simulink model "attitude_modela"  (R2021a)
settings: Solver=VariableStepAuto  StartTime=0.0  StopTime=2000  MaxStep=200
InitFcn:
  | run('parameters.m')
StartFcn:
  | run('parameters.m')
values from neighbouring files (symbols this model uses):
  ARW = (1/4*deg2rad([0.2 0.2 0.2]/sqrt(3600))).^2    [parameters.m]
  c_gyro = 2*sqrt(k*Jz)    [parameters.m]
  Ir = 1e-2    (= 0.01)    [parameters.m]
  J = [0.09 0 0; 0 0.14 0; 0 0 0.07]    [parameters.m]
  Jz = 2e-2    (= 0.02)    [parameters.m]
  k = 10    [parameters.m]    (also in prova.m = size(IGRF,1))
  m_par = [.1 .1 .1]    [parameters.m]
  mu = 398600    [parameters.m]
  nt0 = 0    [parameters.m]
  par = [40073 e deg2rad(59.2548) deg2rad(50) deg2rad(280)]    [parameters.m]
  RRW = (1/4*deg2rad([0.3 0.3 0.3]/3600)).^2    [parameters.m]
  Sch =     [IGRF.mat]
  tsg = 1e-1    (= 0.1)    [parameters.m]
  wr = 100*pi/180    (= 1.74532925199)    [parameters.m]
undefined symbols (not defined in the file or in its folder): DiscIntNeverNeededParam, solar_par
libraries: dspmathops x1, pid_lib x1
settings Model: Creator=matte  LastModifiedBy=simon

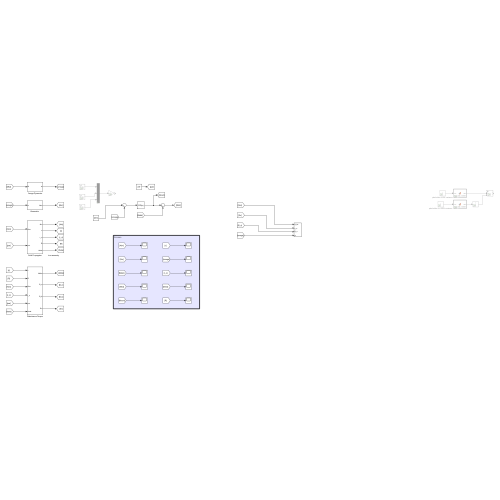
[thumbnail: Simulink's stored preview of the top-level diagram]
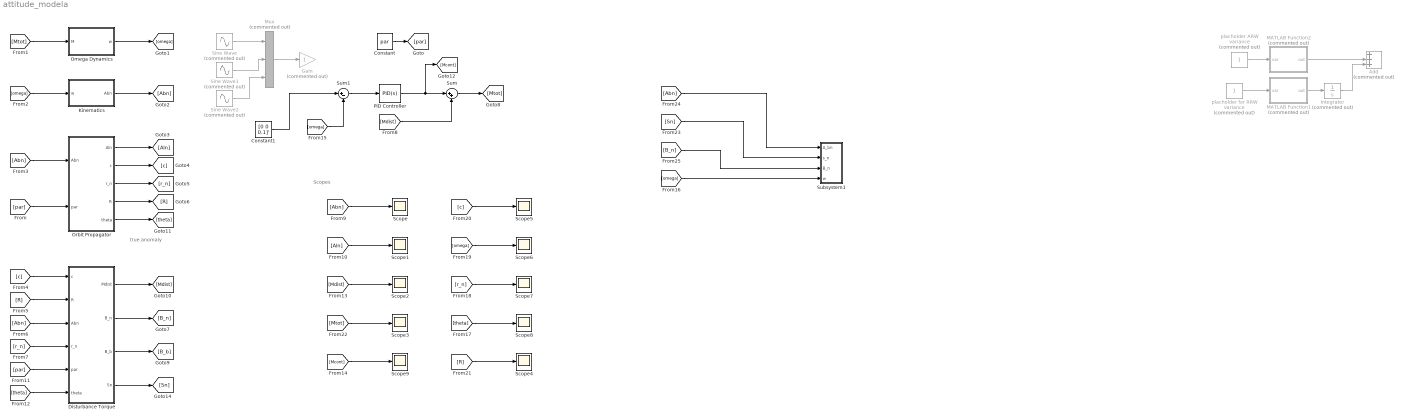
== system attitude_modela ==
  note: Scopes
  note: true anomaly
  Add : Sum  Commented=on  Inputs=+++
  Constant : Constant  Value=par
  Constant1 : Constant  Value=[0 0 0.1]'
  Disturbance Torque : Subsystem
  Gain : Gain  Commented=on
  Integrator : Integrator  Commented=on
  Kinematics : Subsystem
  MATLAB Function1 : MATLAB Function  Commented=on  TreatAsAtomicUnit=on
  MATLAB Function2 : MATLAB Function  Commented=on  TreatAsAtomicUnit=on
  Mux : Mux  Commented=on  Inputs=3
  Omega Dynamics : Subsystem
  Orbit Propagator : Subsystem
  PID Controller : pid_lib/PID Controller  Controller=PID  Form=Parallel  TimeDomain=Continuous-time  UseExternalTs=off  SampleTime=-1  IntegratorMethod=Forward Euler  FilterMethod=Forward Euler  ControllerParametersSource=internal  P=0.1  I=0.01  D=0  UseFilter=on  N=100  TunerSelectOption=Transfer Function Based (PID Tuner App)  InitialConditionSource=internal  InitialConditionForIntegrator=0  InitialConditionForFilter=0  DifferentiatorICPrevScaledInput=0  ExternalReset=none  TrackingMode=off  Kt=1  LimitOutput=off  SatLimitsSource=internal  UpperSaturationLimit=inf  LowerSaturationLimit=-inf  LinearizeAsGain=on  AntiWindupMode=none  Kb=1  POutMin=[]  POutMax=[]  IOutMin=[]  IOutMax=[]  DOutMin=[]  DOutMax=[]  NOutMin=[]  NOutMax=[]  SumOutMin=[]  SumOutMax=[]  SaturationOutMin=[]  SaturationOutMax=[]  PParamMin=[]  PParamMax=[]  IParamMin=[]  IParamMax=[]  DParamMin=[]  DParamMax=[]  NParamMin=[]  NParamMax=[]  KbParamMin=[]  KbParamMax=[]  KtParamMin=[]  KtParamMax=[]  KbOutMin=[]  KbOutMax=[]  KtOutMin=[]  KtOutMax=[]  IntegratorOutMin=[]  IntegratorOutMax=[]  FilterOutMin=[]  FilterOutMax=[]  SumI1OutMin=[]  SumI1OutMax=[]  SumI2OutMin=[]  SumI2OutMax=[]  SumI3OutMin=[]  SumI3OutMax=[]  SumI4OutMin=[]  SumI4OutMax=[]  SumDOutMin=[]  SumDOutMax=[]  DifferentiatorOutMin=[]  DifferentiatorOutMax=[]  FilterDiffOutCoefMin=[]  FilterDiffOutCoefMax=[]  ReciprocalOutMin=[]  ReciprocalOutMax=[]  SumDenOutMin=[]  SumDenOutMax=[]  SumNumOutMin=[]  SumNumOutMax=[]  DivideOutMin=[]  DivideOutMax=[]  UdiffTsProdOutMin=[]  UdiffTsProdOutMax=[]  NTsProdOutMin=[]  NTsProdOutMax=[]  UintegralTsProdOutMin=[]  UintegralTsProdOutMax=[]  UngainTsProdOutMin=[]  UngainTsProdOutMax=[]  IntegratorContinuousStateAttributes=''  IntegratorStateMustResolveToSignalObject=off  IntegratorRTWStateStorageClass=Auto  FilterContinuousStateAttributes=''  FilterStateMustResolveToSignalObject=off  FilterRTWStateStorageClass=Auto  ParallelPVariant=InternalParameters  IdealPVariant=Disabled  IVariant=InternalParameters  DVariant=InternalParameters  IntegratorVariant=Continuous  SatVariant=Disabled  AWVariant=Passthrough  PCopyVariant=Disabled  TRVariant=Disabled  FdbkBlocksVariant=Forward  IdealPFdbkVariant=Disabled  SatFdbkVariant=Disabled  DerivativeFilterVariant=ContFilter  NVariant=InternalParameters  NCopyVariant=Disabled  FilterICVariant=InternalICsFilter  IntegratorICVariant=InternalICs  ExternalResetVariant=Disabled  TRSumVariant=Passthrough  SumFdbkVariant=Disabled  SumVariant=Sum_PID  TsampFilterVariant=InternalTs  TsampNgainVariant=Passthrough  TsampIntegralVariant=Passthrough  ExternalSaturationOutDataTypeStr=Inherit: Same as second input
  Scope{,1..9} (10 alike) : Scope
  Sine Wave : Sin  Commented=on  Amplitude=3  Frequency=2*pi*1e-3  SampleTime=0
  Sine Wave1 : Sin  Commented=on  Amplitude=0.5  Frequency=2*pi*5e-4*0  SampleTime=0
  Sine Wave2 : Sin  Commented=on  Amplitude=0.01  Frequency=2*pi*1e-3  SampleTime=0
  Subsystem1 : Subsystem
  Sum : Sum  Inputs=|++
  Sum1 : Sum  Inputs=|+-
  placholder ARW variance : Constant  Commented=on
  placholder for RRW variance : Constant  Commented=on
  wires:
  Constant/1 -> [par]
  [par] -> Orbit Propagator/2(par)
  PID Controller/1 -> [Mcont], Sum/1
  [Mtot] -> Omega Dynamics/1(M)
  Omega Dynamics/1(w) -> [omega]
  [omega] -> Kinematics/1(w)
  Kinematics/1(Abn) -> [Abn]
  [Abn] -> Orbit Propagator/1(Abn)
  Orbit Propagator/4(R) -> [R]
  Orbit Propagator/3(r_n) -> [r_n]
  Orbit Propagator/2(c) -> [c]
  Orbit Propagator/1(Aln) -> [Aln]
  [Mdist] -> Sum/2
  Sum/1 -> [Mtot]
  Orbit Propagator/5(theta) -> [theta]
  [c] -> Disturbance Torque/1(c)
  [R] -> Disturbance Torque/2(R)
  [Abn] -> Disturbance Torque/3(Abn)
  [r_n] -> Disturbance Torque/4(r_n)
  [par] -> Disturbance Torque/5(par)
  [theta] -> Disturbance Torque/6(theta)
  Disturbance Torque/1(Mdist) -> [Mdist]
  [Abn] -> Scope/1
  [Mdist] -> Scope2/1
  [R] -> Scope4/1
  [omega] -> Scope6/1
  [theta] -> Scope8/1
  [r_n] -> Scope7/1
  [c] -> Scope5/1
  [Mtot] -> Scope3/1
  [Aln] -> Scope1/1
  Disturbance Torque/2(B_n) -> [B_n]
  Disturbance Torque/3(B_b) -> [B_b]
  [Mcont] -> Scope9/1
  MATLAB Function1/1(out) -> Integrator/1
  Integrator/1 -> Add/3
  MATLAB Function2/1(out) -> Add/2
  placholder ARW variance/1 -> MATLAB Function2/1(var)
  placholder for RRW variance/1 -> MATLAB Function1/1(var)
  Disturbance Torque/4(Sn) -> [Sn]
  [omega] -> Sum1/2
  Sum1/1 -> PID Controller/1
  Sine Wave/1 -> Mux/1
  Sine Wave1/1 -> Mux/2
  Sine Wave2/1 -> Mux/3
  Mux/1 -> Gain/1
  [Abn] -> Subsystem1/1(A_bn)
  [Sn] -> Subsystem1/2(s_n)
  [B_n] -> Subsystem1/3(B_n)
  [omega] -> Subsystem1/4(w)
  Constant1/1 -> Sum1/1

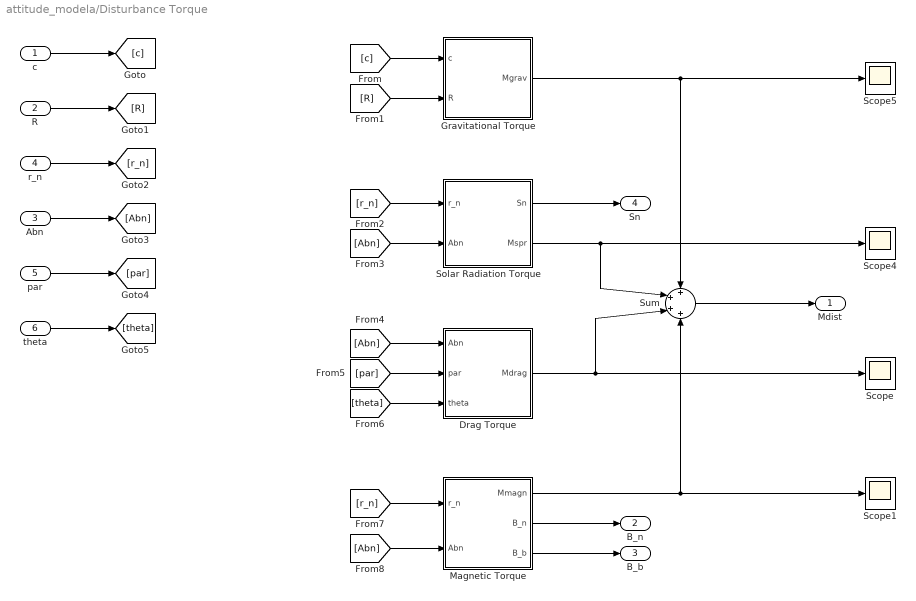
== system attitude_modela/Disturbance Torque ==
  c : Inport
  R : Inport  Port=2
  Abn : Inport  Port=3
  r_n : Inport  Port=4
  par : Inport  Port=5
  theta : Inport  Port=6
  Drag Torque : Subsystem
  Gravitational Torque : Subsystem
  Magnetic Torque : Subsystem
  Scope{,1,4..5} (4 alike) : Scope
  Solar Radiation Torque : Subsystem
  Sum : Sum  Inputs=4
  Mdist : Outport
  B_n : Outport  Port=2
  B_b : Outport  Port=3
  Sn : Outport  Port=4
  wires:
  Sum/1 -> Mdist/1
  Magnetic Torque/2(B_n) -> B_n/1
  Magnetic Torque/3(B_b) -> B_b/1
  c/1 -> [c]
  R/1 -> [R]
  r_n/1 -> [r_n]
  Abn/1 -> [Abn]
  par/1 -> [par]
  theta/1 -> [theta]
  Magnetic Torque/1(Mmagn) -> Scope1/1, Sum/4
  Drag Torque/1(Mdrag) -> Sum/3, Scope/1
  Solar Radiation Torque/2(Mspr) -> Scope4/1, Sum/2
  Gravitational Torque/1(Mgrav) -> Scope5/1, Sum/1
  [Abn] -> Magnetic Torque/2(Abn)
  [r_n] -> Magnetic Torque/1(r_n)
  [Abn] -> Drag Torque/1(Abn)
  [par] -> Drag Torque/2(par)
  [theta] -> Drag Torque/3(theta)
  [Abn] -> Solar Radiation Torque/2(Abn)
  [r_n] -> Solar Radiation Torque/1(r_n)
  [R] -> Gravitational Torque/2(R)
  [c] -> Gravitational Torque/1(c)
  Solar Radiation Torque/1(Sn) -> Sn/1

== system attitude_modela/Kinematics ==
  w : Inport
  Gain : Gain  Gain=-1
  Integrator : Integrator  InitialCondition=eye(3)
  Levi-Civita Matrix : Subsystem
  Product : Product  Multiplication=Matrix(*)
  Subsystem : Subsystem
  Abn : Outport
  wires:
  Product/1 -> Gain/1
  Levi-Civita Matrix/1(w^) -> Product/1
  w/1 -> Levi-Civita Matrix/1(w)
  Gain/1 -> Integrator/1  "dA"
  Integrator/1 -> Subsystem/1(A0)
  Subsystem/1(A) -> Abn/1, Product/2

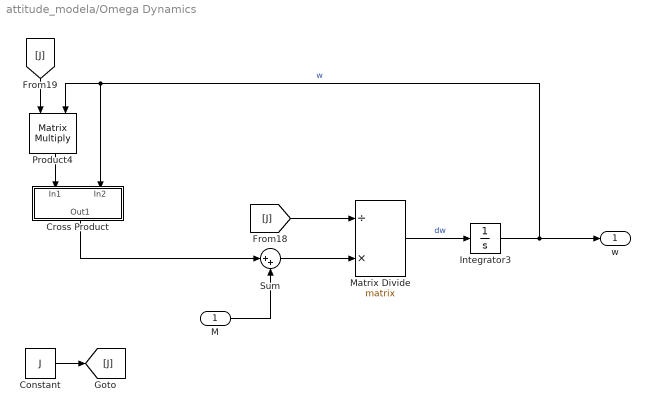
== system attitude_modela/Omega Dynamics ==
  M : Inport
  Constant : Constant  Value=J
  Cross Product : Subsystem  Description=Replaced Block  mask(Replaced Block){}
      mask help: This block has been replaced with an empty subsystem because it used functionality that is unavailable in Simulink R2021a.
      mask Display: fprintf('Replaced: %s\n','CrossProduct')
  Integrator3 : Integrator  InitialCondition=zeros(3,1)
  Matrix Divide : Product  Inputs=/*  Multiplication=Matrix(*)
  Product4 : Product  Multiplication=Matrix(*)
  Sum : Sum  Inputs=|++
  w : Outport
  wires:
  M/1 -> Sum/2
  Matrix Divide/1 -> Integrator3/1  "dw"
  Product4/1 -> Cross Product/1(In1)
  Integrator3/1 -> w/1, Product4/2, Cross Product/2(In2)  "w"
  Constant/1 -> [J]
  [J] -> Matrix Divide/1
  [J] -> Product4/1
  Cross Product/1(Out1) -> Sum/1
  Sum/1 -> Matrix Divide/2

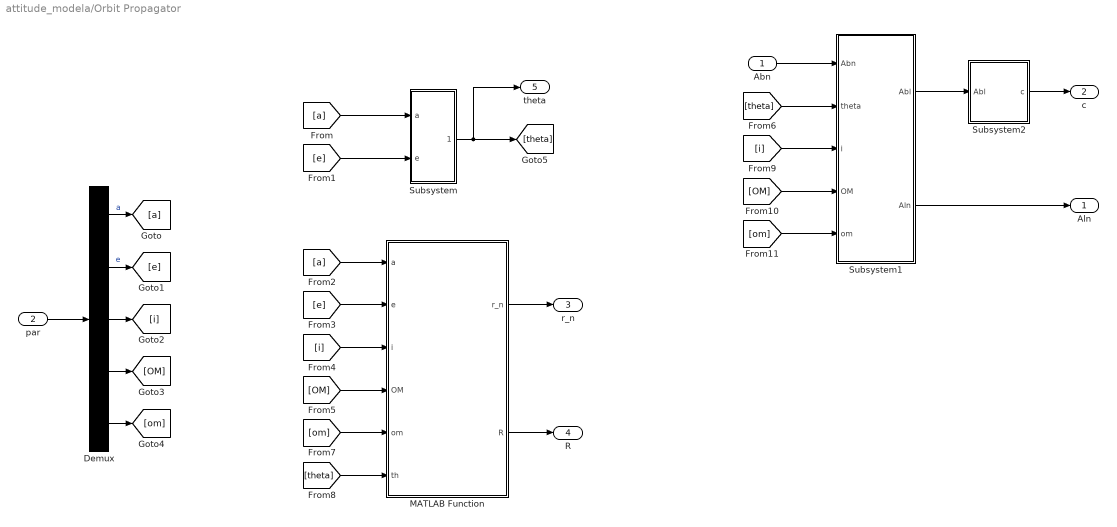
== system attitude_modela/Orbit Propagator ==
  Abn : Inport
  par : Inport  Port=2
  Demux : Demux  Outputs=5
  MATLAB Function : MATLAB Function  TreatAsAtomicUnit=on
  Subsystem : Subsystem
  Subsystem1 : Subsystem
  Subsystem2 : Subsystem
  Aln : Outport
  c : Outport  Port=2
  r_n : Outport  Port=3
  R : Outport  Port=4
  theta : Outport  Port=5
  wires:
  Abn/1 -> Subsystem1/1(Abn)
  Subsystem1/1(Abl) -> Subsystem2/1(Abl)
  Subsystem1/2(Aln) -> Aln/1
  par/1 -> Demux/1
  Subsystem2/1(c) -> c/1
  Demux/1 -> [a]  "a"
  Demux/2 -> [e]  "e"
  Demux/3 -> [i]
  Demux/4 -> [OM]
  Demux/5 -> [om]
  [e] -> MATLAB Function/2(e)
  [a] -> MATLAB Function/1(a)
  [OM] -> MATLAB Function/4(OM)
  [i] -> MATLAB Function/3(i)
  [theta] -> Subsystem1/2(theta)
  Subsystem/1(theta) -> theta/1, [theta]
  [om] -> MATLAB Function/5(om)
  [theta] -> MATLAB Function/6(th)
  MATLAB Function/1(r_n) -> r_n/1
  MATLAB Function/2(R) -> R/1
  [i] -> Subsystem1/3(i)
  [OM] -> Subsystem1/4(OM)
  [om] -> Subsystem1/5(om)
  [e] -> Subsystem/2(e)
  [a] -> Subsystem/1(a)

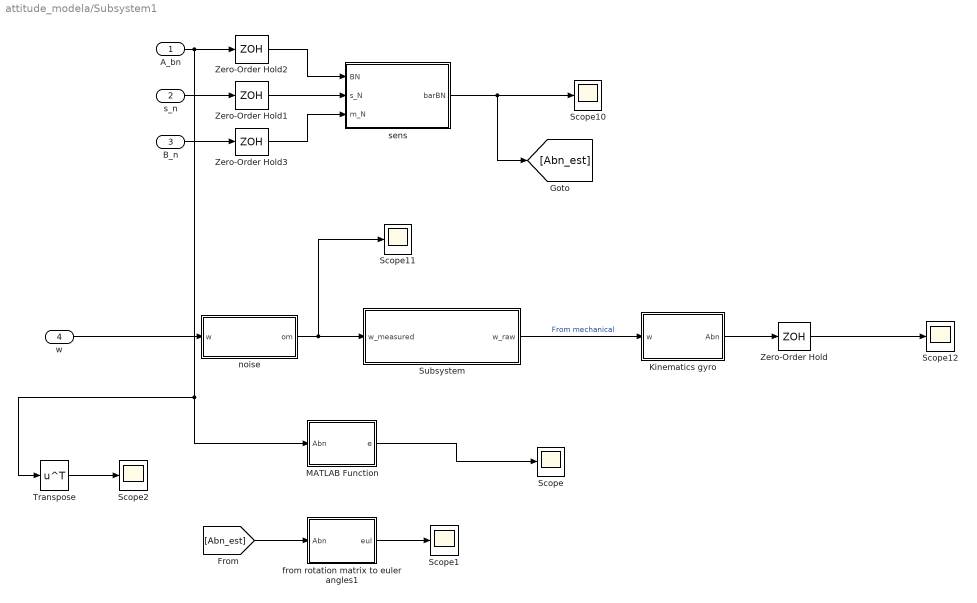
== system attitude_modela/Subsystem1 ==
  A_bn : Inport
  s_n : Inport  Port=2
  B_n : Inport  Port=3
  w : Inport  Port=4
  Kinematics gyro : Subsystem
  MATLAB Function : MATLAB Function  TreatAsAtomicUnit=on
  Scope{,1..2,10..12} (6 alike) : Scope
  Subsystem : Subsystem
  Transpose : Math  Operator=transpose  SaturateOnIntegerOverflow=on
  Zero-Order Hold{,1..3} (4 alike) : ZeroOrderHold  SampleTime=tsg
  from rotation matrix to euler angles1 : MATLAB Function  TreatAsAtomicUnit=on
  noise : Subsystem
  sens : MATLAB Function  TreatAsAtomicUnit=on
  wires:
  Zero-Order Hold/1 -> Scope12/1
  B_n/1 -> Zero-Order Hold3/1
  Kinematics gyro/1(Abn) -> Zero-Order Hold/1
  Subsystem/1(w_raw) -> Kinematics gyro/1(w)  "From mechanical"
  Zero-Order Hold1/1 -> sens/2(s_N)
  noise/1(om) -> Scope11/1, Subsystem/1(w_measured)
  Zero-Order Hold3/1 -> sens/3(m_N)
  sens/1(barBN) -> [Abn_est], Scope10/1
  w/1 -> noise/1(w)
  s_n/1 -> Zero-Order Hold1/1
  A_bn/1 -> Transpose/1, MATLAB Function/1(Abn), Zero-Order Hold2/1
  Zero-Order Hold2/1 -> sens/1(BN)
  [Abn_est] -> from rotation matrix to euler angles1/1(Abn)
  from rotation matrix to euler angles1/1(eul) -> Scope1/1
  MATLAB Function/1(e) -> Scope/1
  Transpose/1 -> Scope2/1

== system attitude_modela/Disturbance Torque/Drag Torque ==
  Abn : Inport
  par : Inport  Port=2
  theta : Inport  Port=3
  Drag Torque : MATLAB Function  TreatAsAtomicUnit=on
  Mdrag : Outport
  wires:
  Drag Torque/1(Mdrag) -> Mdrag/1
  Abn/1 -> Drag Torque/1(Abn)
  theta/1 -> Drag Torque/3(theta)
  par/1 -> Drag Torque/2(par)

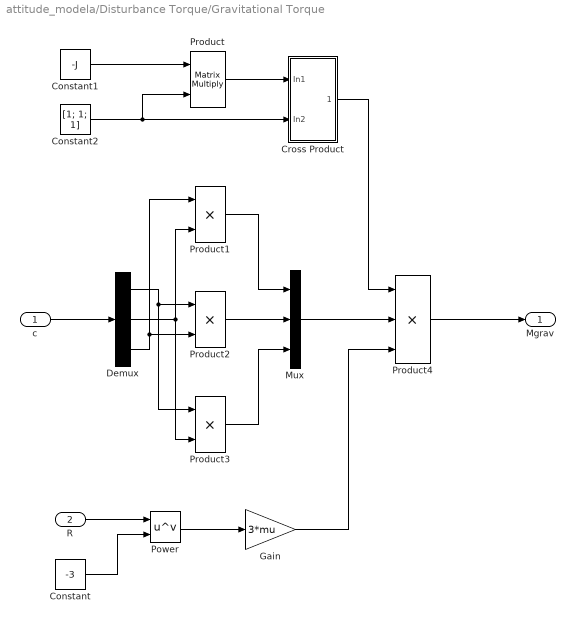
== system attitude_modela/Disturbance Torque/Gravitational Torque ==
  c : Inport
  R : Inport  Port=2
  Constant : Constant  Value=-3
  Constant1 : Constant  Value=-J
  Constant2 : Constant  Value=[1; 1; 1]
  Cross Product : Subsystem  Description=Replaced Block  mask(Replaced Block){}
      mask help: This block has been replaced with an empty subsystem because it used functionality that is unavailable in Simulink R2021a.
      mask Display: fprintf('Replaced: %s\n','CrossProduct')
  Demux : Demux  Outputs=3
  Gain : Gain  Gain=3*mu
  Mux : Mux  Inputs=3
  Power : Math  Operator=pow  SaturateOnIntegerOverflow=on
  Product : Product  Multiplication=Matrix(*)
  Product1 : Product
  Product2 : Product
  Product3 : Product
  Product4 : Product  Inputs=3
  Mgrav : Outport
  wires:
  Constant/1 -> Power/2
  R/1 -> Power/1
  Power/1 -> Gain/1
  Constant1/1 -> Product/1
  Constant2/1 -> Product/2, Cross Product/2(In2)
  Product/1 -> Cross Product/1(In1)
  c/1 -> Demux/1
  Demux/1 -> Product2/1, Product3/1
  Demux/3 -> Product1/1, Product2/2
  Demux/2 -> Product1/2, Product3/2
  Product2/1 -> Mux/2
  Product1/1 -> Mux/1
  Product3/1 -> Mux/3
  Cross Product/1(Out1) -> Product4/1
  Mux/1 -> Product4/2
  Gain/1 -> Product4/3
  Product4/1 -> Mgrav/1

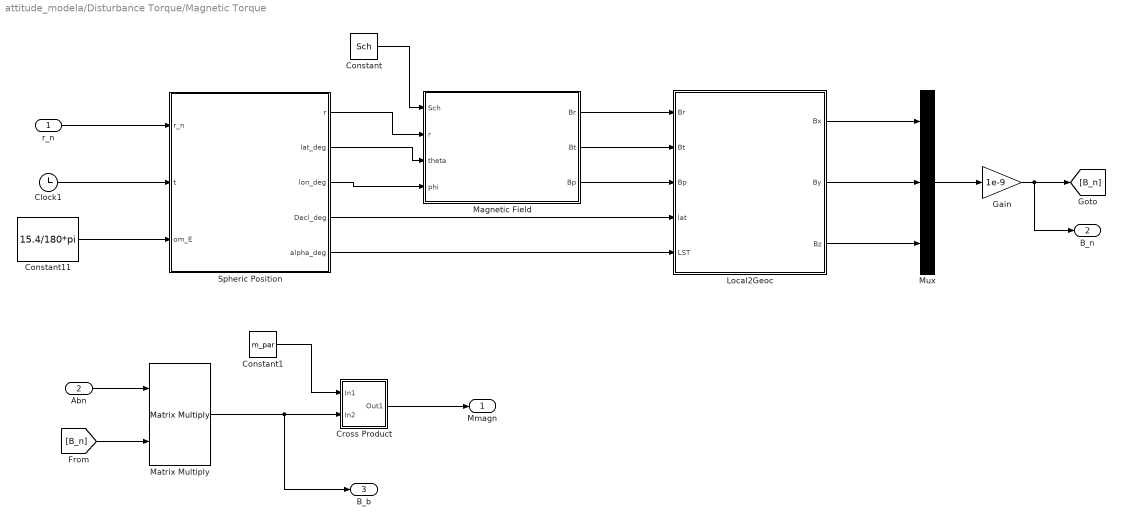
== system attitude_modela/Disturbance Torque/Magnetic Torque ==
  r_n : Inport
  Abn : Inport  Port=2
  Clock1 : Clock
  Constant : Constant  Value=Sch  OutDataTypeStr=Bus: Sch_bus
  Constant1 : Constant  Value=m_par
  Constant11 : Constant  Value=15.4/180*pi
  Cross Product : Subsystem  Description=Replaced Block  mask(Replaced Block){}
      mask help: This block has been replaced with an empty subsystem because it used functionality that is unavailable in Simulink R2021a.
      mask Display: fprintf('Replaced: %s\n','CrossProduct')
  Gain : Gain  Gain=1e-9
  Local2Geoc : MATLAB Function  TreatAsAtomicUnit=on
  Magnetic Field : MATLAB Function  TreatAsAtomicUnit=on
  Matrix Multiply : Product  Multiplication=Matrix(*)
  Mux : Mux  Inputs=3
  Spheric Position : MATLAB Function  TreatAsAtomicUnit=on
  Mmagn : Outport
  B_n : Outport  Port=2
  B_b : Outport  Port=3
  wires:
  r_n/1 -> Spheric Position/1(r_n)
  Constant11/1 -> Spheric Position/3(om_E)
  Clock1/1 -> Spheric Position/2(t)
  Spheric Position/1(r) -> Magnetic Field/2(r)
  Spheric Position/2(lat_deg) -> Magnetic Field/3(theta)
  Spheric Position/3(lon_deg) -> Magnetic Field/4(phi)
  Magnetic Field/1(Br) -> Local2Geoc/1(Br)
  Magnetic Field/2(Bt) -> Local2Geoc/2(Bt)
  Magnetic Field/3(Bp) -> Local2Geoc/3(Bp)
  Spheric Position/4(Decl_deg) -> Local2Geoc/4(lat)
  Spheric Position/5(alpha_deg) -> Local2Geoc/5(LST)
  Local2Geoc/1(Bx) -> Mux/1
  Local2Geoc/2(By) -> Mux/2
  Local2Geoc/3(Bz) -> Mux/3
  Mux/1 -> Gain/1
  Constant/1 -> Magnetic Field/1(Sch)
  Gain/1 -> B_n/1, [B_n]
  Abn/1 -> Matrix Multiply/1
  [B_n] -> Matrix Multiply/2
  Constant1/1 -> Cross Product/1(In1)
  Cross Product/1(Out1) -> Mmagn/1
  Matrix Multiply/1 -> B_b/1, Cross Product/2(In2)

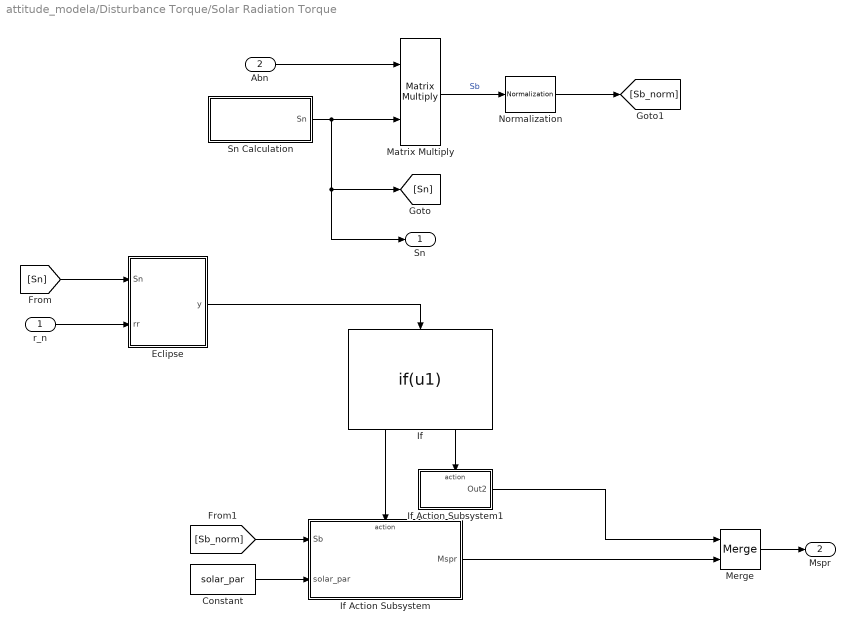
== system attitude_modela/Disturbance Torque/Solar Radiation Torque ==
  r_n : Inport
  Abn : Inport  Port=2
  Constant : Constant  Value=solar_par  OutDataTypeStr=Bus: solar_par_bus
  Eclipse : MATLAB Function  TreatAsAtomicUnit=on
  If : If  IfExpression=u1
  If Action Subsystem : Subsystem  TreatAsAtomicUnit=on
  If Action Subsystem1 : Subsystem  TreatAsAtomicUnit=on
  Matrix Multiply : Product  Multiplication=Matrix(*)
  Merge : Merge
  Normalization : dspmathops/Normalization  NormType=Squared 2-norm  Bias=1e-10  NormOver=Each column  Dimension=1  roundingMode=Floor  overflowMode=off  accumDataTypeStr=Inherit: Same as product output  accumLastDataTypeStr=Inherit: Same as product output  outputDataTypeStr=Inherit: Same as product output  outputMin=[]  outputMax=[]  outputLastDataTypeStr=Inherit: Same as product output
  Sn Calculation : Subsystem
  Sn : Outport
  Mspr : Outport  Port=2
  wires:
  Sn Calculation/1(Sn) -> Sn/1, [Sn], Matrix Multiply/2
  Abn/1 -> Matrix Multiply/1
  r_n/1 -> Eclipse/2(rr)
  [Sn] -> Eclipse/1(Sn)
  Matrix Multiply/1 -> Normalization/1  "Sb"
  Normalization/1 -> [Sb_norm]
  If/1 -> If Action Subsystem/Action
  [Sb_norm] -> If Action Subsystem/1(Sb)
  Constant/1 -> If Action Subsystem/2(solar_par)
  Merge/1 -> Mspr/1
  If/2 -> If Action Subsystem1/Action
  If Action Subsystem/1(Mspr) -> Merge/2
  If Action Subsystem1/1(Out2) -> Merge/1
  Eclipse/1(y) -> If/1

== system attitude_modela/Kinematics/Levi-Civita Matrix ==
  w : Inport
  Constant : Constant  Value=[0; 0; 1]
  Constant1 : Constant  Value=[0; 1; 0]
  Constant2 : Constant  Value=[1; 0; 0]
  Cross Product : Subsystem  Description=Replaced Block  mask(Replaced Block){}
      mask help: This block has been replaced with an empty subsystem because it used functionality that is unavailable in Simulink R2021a.
      mask Display: fprintf('Replaced: %s\n','CrossProduct')
  Cross Product1 : Subsystem  Description=Replaced Block  mask(Replaced Block){}
      mask help: This block has been replaced with an empty subsystem because it used functionality that is unavailable in Simulink R2021a.
      mask Display: fprintf('Replaced: %s\n','CrossProduct')
  Cross Product2 : Subsystem  Description=Replaced Block  mask(Replaced Block){}
      mask help: This block has been replaced with an empty subsystem because it used functionality that is unavailable in Simulink R2021a.
      mask Display: fprintf('Replaced: %s\n','CrossProduct')
  Matrix Concatenate : Concatenate  NumInputs=3  Mode=Multidimensional array  ConcatenateDimension=2
  w^ : Outport
  wires:
  Constant2/1 -> Cross Product/2(In2)
  Constant/1 -> Cross Product2/2(In2)
  Cross Product/1(Out1) -> Matrix Concatenate/1
  Cross Product2/1(Out1) -> Matrix Concatenate/3
  Constant1/1 -> Cross Product1/2(In2)
  Cross Product1/1(Out1) -> Matrix Concatenate/2
  Matrix Concatenate/1 -> w^/1
  w/1 -> Cross Product/1(In1), Cross Product2/1(In1), Cross Product1/1(In1)

== system attitude_modela/Kinematics/Subsystem ==
  A0 : Inport
  Add : Sum  Inputs=+-
  Gain : Gain  Gain=1.5
  Gain1 : Gain  Gain=0.5
  Product1 : Product  Inputs=3  Multiplication=Matrix(*)
  Transpose : Math  Operator=transpose  SaturateOnIntegerOverflow=on
  A : Outport
  wires:
  Add/1 -> A/1
  Gain/1 -> Add/1
  A0/1 -> Product1/1, Gain1/1, Transpose/1, Gain/1
  Transpose/1 -> Product1/2
  Product1/1 -> Add/2
  Gain1/1 -> Product1/3

== system attitude_modela/Omega Dynamics/Cross Product ==
  In1 : Inport
  In2 : Inport  Port=2
  Ground1 : Ground
  Terminator1 : Terminator
  Terminator2 : Terminator
  Out1 : Outport
  wires:
  Ground1/1 -> Out1/1
  In2/1 -> Terminator2/1
  In1/1 -> Terminator1/1

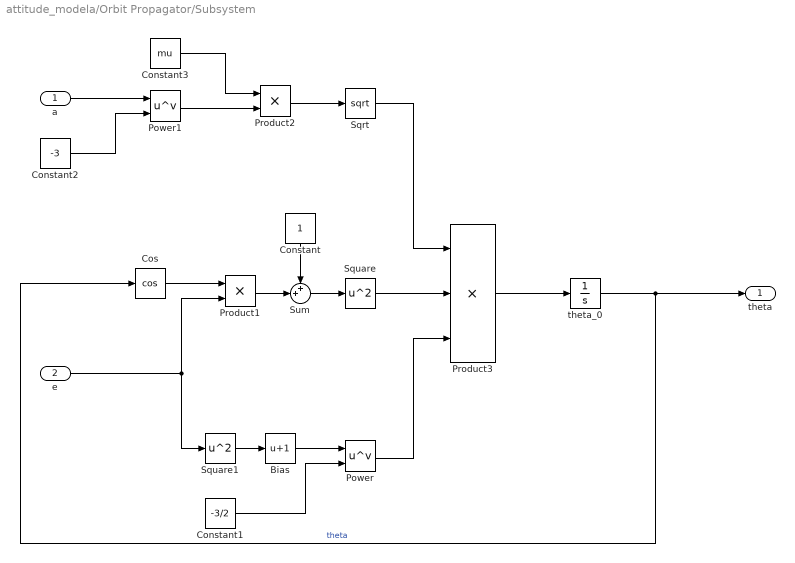
== system attitude_modela/Orbit Propagator/Subsystem ==
  a : Inport
  e : Inport  Port=2
  Bias : Bias  Bias=1
  Constant : Constant
  Constant1 : Constant  Value=-3/2
  Constant2 : Constant  Value=-3
  Constant3 : Constant  Value=mu
  Cos : Trigonometry  Operator=cos
  Power : Math  Operator=pow  SaturateOnIntegerOverflow=on
  Power1 : Math  Operator=pow  SaturateOnIntegerOverflow=on
  Product1 : Product
  Product2 : Product
  Product3 : Product  Inputs=3
  Sqrt : Sqrt  SaturateOnIntegerOverflow=on
  Square : Math  Operator=square  SaturateOnIntegerOverflow=on
  Square1 : Math  Operator=square  SaturateOnIntegerOverflow=on
  Sum : Sum  Inputs=++|
  theta_0 : Integrator
  theta : Outport
  wires:
  Constant2/1 -> Power1/2
  Power1/1 -> Product2/2
  Product2/1 -> Sqrt/1
  a/1 -> Power1/1
  Constant3/1 -> Product2/1
  Sum/1 -> Square/1
  Product1/1 -> Sum/2
  Constant/1 -> Sum/1
  Constant1/1 -> Power/2
  theta_0/1 -> Cos/1, theta/1  "theta"
  Cos/1 -> Product1/1
  e/1 -> Square1/1, Product1/2
  Square/1 -> Product3/2
  Power/1 -> Product3/3
  Sqrt/1 -> Product3/1
  Product3/1 -> theta_0/1
  Square1/1 -> Bias/1
  Bias/1 -> Power/1

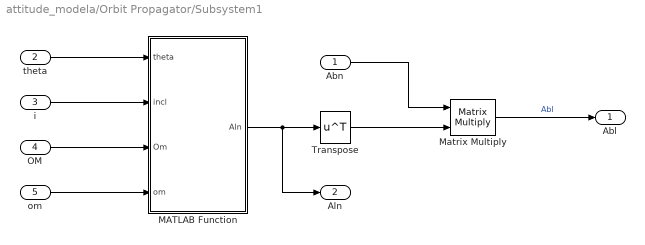
== system attitude_modela/Orbit Propagator/Subsystem1 ==
  Abn : Inport
  theta : Inport  Port=2
  i : Inport  Port=3
  OM : Inport  Port=4
  om : Inport  Port=5
  MATLAB Function : MATLAB Function  TreatAsAtomicUnit=on
  Matrix Multiply : Product  Multiplication=Matrix(*)
  Transpose : Math  Operator=transpose  SaturateOnIntegerOverflow=on
  Abl : Outport
  Aln : Outport  Port=2
  wires:
  Matrix Multiply/1 -> Abl/1  "Abl"
  MATLAB Function/1(Aln) -> Aln/1, Transpose/1
  theta/1 -> MATLAB Function/1(theta)
  Transpose/1 -> Matrix Multiply/2
  Abn/1 -> Matrix Multiply/1
  i/1 -> MATLAB Function/2(incl)
  OM/1 -> MATLAB Function/3(Om)
  om/1 -> MATLAB Function/4(om)

== system attitude_modela/Orbit Propagator/Subsystem2 ==
  Abl : Inport
  Constant : Constant  Value=[1; 0; 0]
  Matrix Multiply1 : Product  Multiplication=Matrix(*)
  c : Outport
  wires:
  Matrix Multiply1/1 -> c/1  "c"
  Abl/1 -> Matrix Multiply1/1  "Abl"
  Constant/1 -> Matrix Multiply1/2

== system attitude_modela/Subsystem1/Kinematics gyro ==
  w : Inport
  Gain : Gain  Gain=-1
  Integrator : Integrator  InitialCondition=eye(3)
  Levi-Civita Matrix : Subsystem
  Product : Product  Multiplication=Matrix(*)
  Subsystem : Subsystem
  Abn : Outport
  wires:
  Subsystem/1(A) -> Product/2, Abn/1
  Integrator/1 -> Subsystem/1(A0)
  Gain/1 -> Integrator/1  "dA"
  w/1 -> Levi-Civita Matrix/1(w)
  Levi-Civita Matrix/1(w^) -> Product/1
  Product/1 -> Gain/1

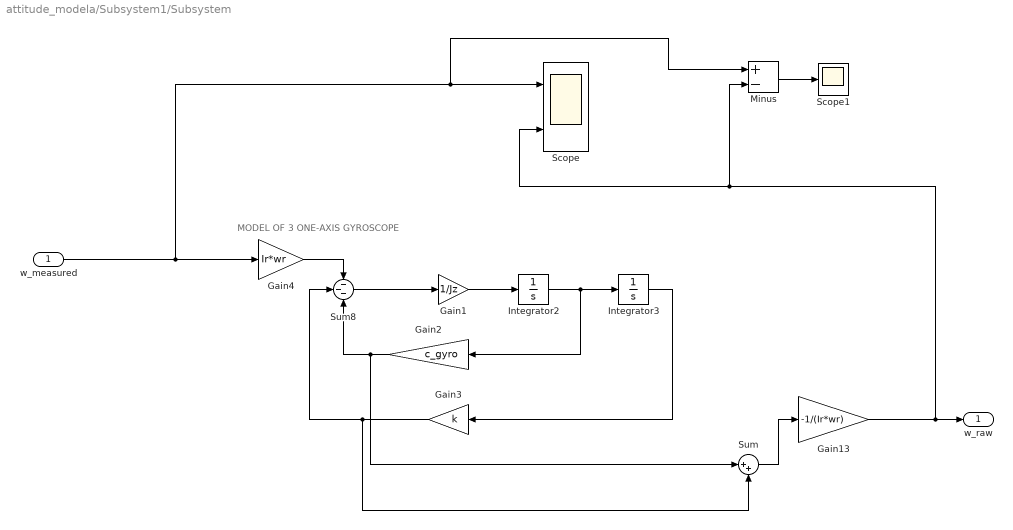
== system attitude_modela/Subsystem1/Subsystem ==
  note: MODEL OF 3 ONE-AXIS GYROSCOPE
  w_measured : Inport
  Gain1 : Gain  Gain=1/Jz
  Gain13 : Gain  Gain=-1/(Ir*wr)
  Gain2 : Gain  Gain=c_gyro
  Gain3 : Gain  Gain=k
  Gain4 : Gain  Gain=Ir*wr
  Integrator2 : Integrator  InitialCondition=[0 0 0]'
  Integrator3 : Integrator  InitialCondition=[0 0 0]'
  Minus : Sum  Inputs=+-
  Scope : Scope  NumInputPorts=2
  Scope1 : Scope
  Sum : Sum  Inputs=|++
  Sum8 : Sum  Inputs=---
  w_raw : Outport
  wires:
  Gain1/1 -> Integrator2/1
  Integrator2/1 -> Gain2/1, Integrator3/1
  Sum8/1 -> Gain1/1
  w_measured/1 -> Minus/1, Scope/1, Gain4/1
  Integrator3/1 -> Gain3/1
  Gain3/1 -> Sum/2, Sum8/2
  Gain2/1 -> Sum/1, Sum8/3
  Gain13/1 -> Minus/2, Scope/2, w_raw/1
  Gain4/1 -> Sum8/1
  Sum/1 -> Gain13/1
  Minus/1 -> Scope1/1

== system attitude_modela/Subsystem1/noise ==
  w : Inport
  ARW : RandomNumber  Variance=ARW  SampleTime=tsg
  Discrete-Time Integrator : DiscreteIntegrator  SampleTime=-1  ICPrevOutput=DiscIntNeverNeededParam  ICPrevScaledInput=DiscIntNeverNeededParam
  RRW : RandomNumber  Variance=RRW  SampleTime=tsg
  Sum : Sum  Inputs=3
  om : Outport
  wires:
  RRW/1 -> Discrete-Time Integrator/1
  w/1 -> Sum/2
  ARW/1 -> Sum/1
  Sum/1 -> om/1
  Discrete-Time Integrator/1 -> Sum/3

== system attitude_modela/Disturbance Torque/Gravitational Torque/Cross Product ==
  In1 : Inport
  In2 : Inport  Port=2
  Ground1 : Ground
  Terminator1 : Terminator
  Terminator2 : Terminator
  Out1 : Outport
  wires:
  Ground1/1 -> Out1/1
  In2/1 -> Terminator2/1
  In1/1 -> Terminator1/1

== system attitude_modela/Disturbance Torque/Magnetic Torque/Cross Product ==
  In1 : Inport
  In2 : Inport  Port=2
  Ground1 : Ground
  Terminator1 : Terminator
  Terminator2 : Terminator
  Out1 : Outport
  wires:
  Ground1/1 -> Out1/1
  In2/1 -> Terminator2/1
  In1/1 -> Terminator1/1

== system attitude_modela/Disturbance Torque/Solar Radiation Torque/If Action Subsystem ==
  Sb : Inport
  solar_par : Inport  Port=2
  Action Port : ActionPort  ActionPortLabel=if(u1)
  Torque Compute : MATLAB Function  TreatAsAtomicUnit=on
  Mspr : Outport
  wires:
  Torque Compute/1(Mspr) -> Mspr/1  "Mspr"
  Sb/1 -> Torque Compute/1(Sb)
  solar_par/1 -> Torque Compute/2(solar_par)

== system attitude_modela/Disturbance Torque/Solar Radiation Torque/If Action Subsystem1 ==
  Action Port : ActionPort  ActionPortLabel=else
  Constant1 : Constant  Value=[0 0 0]
  Out2 : Outport
  wires:
  Constant1/1 -> Out2/1

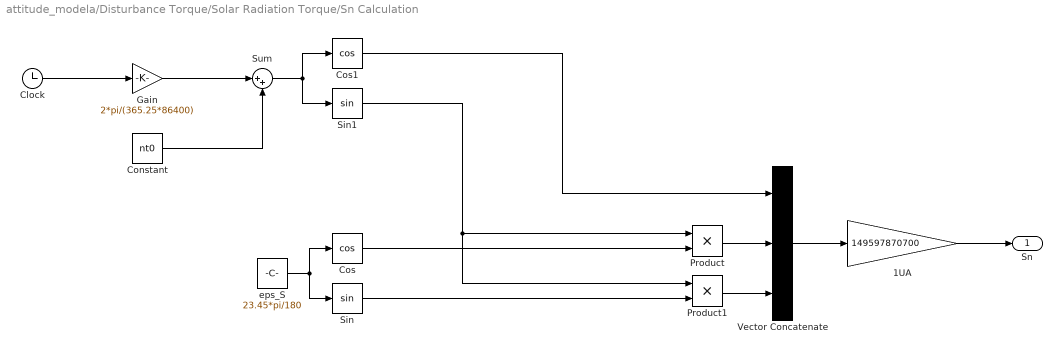
== system attitude_modela/Disturbance Torque/Solar Radiation Torque/Sn Calculation ==
  1UA : Gain  Gain=149597870700
  Clock : Clock
  Constant : Constant  Value=nt0
  Cos : Trigonometry  Operator=cos
  Cos1 : Trigonometry  Operator=cos
  Gain : Gain  Gain=2*pi/(365.25*86400)
  Product : Product
  Product1 : Product
  Sin : Trigonometry
  Sin1 : Trigonometry
  Sum : Sum  Inputs=|++
  Vector Concatenate : Concatenate  NumInputs=3
  eps_S : Constant  Value=23.45*pi/180
  Sn : Outport
  wires:
  Vector Concatenate/1 -> 1UA/1
  1UA/1 -> Sn/1
  Gain/1 -> Sum/1
  Clock/1 -> Gain/1
  Constant/1 -> Sum/2
  Product/1 -> Vector Concatenate/2
  Product1/1 -> Vector Concatenate/3
  eps_S/1 -> Cos/1, Sin/1
  Cos/1 -> Product/2
  Sin/1 -> Product1/2
  Sum/1 -> Sin1/1, Cos1/1
  Cos1/1 -> Vector Concatenate/1
  Sin1/1 -> Product1/1, Product/1

== system attitude_modela/Kinematics/Levi-Civita Matrix/Cross Product ==
  In1 : Inport
  In2 : Inport  Port=2
  Ground1 : Ground
  Terminator1 : Terminator
  Terminator2 : Terminator
  Out1 : Outport
  wires:
  Ground1/1 -> Out1/1
  In2/1 -> Terminator2/1
  In1/1 -> Terminator1/1

== system attitude_modela/Kinematics/Levi-Civita Matrix/Cross Product1 ==
  In1 : Inport
  In2 : Inport  Port=2
  Ground1 : Ground
  Terminator1 : Terminator
  Terminator2 : Terminator
  Out1 : Outport
  wires:
  Ground1/1 -> Out1/1
  In2/1 -> Terminator2/1
  In1/1 -> Terminator1/1

== system attitude_modela/Kinematics/Levi-Civita Matrix/Cross Product2 ==
  In1 : Inport
  In2 : Inport  Port=2
  Ground1 : Ground
  Terminator1 : Terminator
  Terminator2 : Terminator
  Out1 : Outport
  wires:
  Ground1/1 -> Out1/1
  In2/1 -> Terminator2/1
  In1/1 -> Terminator1/1

== system attitude_modela/Subsystem1/Kinematics gyro/Levi-Civita Matrix ==
  w : Inport
  Constant : Constant  Value=[0; 0; 1]
  Constant1 : Constant  Value=[0; 1; 0]
  Constant2 : Constant  Value=[1; 0; 0]
  Cross Product : Subsystem  Description=Replaced Block  mask(Replaced Block){}
      mask help: This block has been replaced with an empty subsystem because it used functionality that is unavailable in Simulink R2021a.
      mask Display: fprintf('Replaced: %s\n','CrossProduct')
  Cross Product1 : Subsystem  Description=Replaced Block  mask(Replaced Block){}
      mask help: This block has been replaced with an empty subsystem because it used functionality that is unavailable in Simulink R2021a.
      mask Display: fprintf('Replaced: %s\n','CrossProduct')
  Cross Product2 : Subsystem  Description=Replaced Block  mask(Replaced Block){}
      mask help: This block has been replaced with an empty subsystem because it used functionality that is unavailable in Simulink R2021a.
      mask Display: fprintf('Replaced: %s\n','CrossProduct')
  Matrix Concatenate : Concatenate  NumInputs=3  Mode=Multidimensional array  ConcatenateDimension=2
  w^ : Outport
  wires:
  w/1 -> Cross Product1/1(In1), Cross Product2/1(In1), Cross Product/1(In1)
  Matrix Concatenate/1 -> w^/1
  Cross Product1/1(Out1) -> Matrix Concatenate/2
  Constant1/1 -> Cross Product1/2(In2)
  Cross Product2/1(Out1) -> Matrix Concatenate/3
  Cross Product/1(Out1) -> Matrix Concatenate/1
  Constant/1 -> Cross Product2/2(In2)
  Constant2/1 -> Cross Product/2(In2)

== system attitude_modela/Subsystem1/Kinematics gyro/Subsystem ==
  A0 : Inport
  Add : Sum  Inputs=+-
  Gain : Gain  Gain=1.5
  Gain1 : Gain  Gain=0.5
  Product1 : Product  Inputs=3  Multiplication=Matrix(*)
  Transpose : Math  Operator=transpose  SaturateOnIntegerOverflow=on
  A : Outport
  wires:
  Gain1/1 -> Product1/3
  Product1/1 -> Add/2
  Transpose/1 -> Product1/2
  A0/1 -> Gain/1, Transpose/1, Gain1/1, Product1/1
  Gain/1 -> Add/1
  Add/1 -> A/1

== system attitude_modela/Subsystem1/Kinematics gyro/Levi-Civita Matrix/Cross Product ==
  In1 : Inport
  In2 : Inport  Port=2
  Ground1 : Ground
  Terminator1 : Terminator
  Terminator2 : Terminator
  Out1 : Outport
  wires:
  Ground1/1 -> Out1/1
  In2/1 -> Terminator2/1
  In1/1 -> Terminator1/1

== system attitude_modela/Subsystem1/Kinematics gyro/Levi-Civita Matrix/Cross Product1 ==
  In1 : Inport
  In2 : Inport  Port=2
  Ground1 : Ground
  Terminator1 : Terminator
  Terminator2 : Terminator
  Out1 : Outport
  wires:
  Ground1/1 -> Out1/1
  In2/1 -> Terminator2/1
  In1/1 -> Terminator1/1

== system attitude_modela/Subsystem1/Kinematics gyro/Levi-Civita Matrix/Cross Product2 ==
  In1 : Inport
  In2 : Inport  Port=2
  Ground1 : Ground
  Terminator1 : Terminator
  Terminator2 : Terminator
  Out1 : Outport
  wires:
  Ground1/1 -> Out1/1
  In2/1 -> Terminator2/1
  In1/1 -> Terminator1/1

== matlab function attitude_modela/Disturbance Torque/Magnetic Torque/Spheric Position ==
  data: r output; lat_deg output; r_n input; lon_deg output; t input; Decl_deg output; alpha_deg output; om_E input
function [r,lat_deg,lon_deg,Decl_deg,alpha_deg] = spheric(r_n,t,om_E)
t0=0;
Rp=om_E;
r=norm(r_n);
Decl=asin(r_n(3)/r);             %Calculating the declination
if r_n(2)/r>0                                                          %Calculating the right ascension
    alpha=acos((r_n(1)/r)/cos(Decl));
else
    alpha=2*pi-acos((r_n(1)/r)/cos(Decl));
end
ThetaG=Rp.*(t-t0)./3600; %Calculating the vector of position of the Greenwich Parallel NOTE: Rp=[Rad/h]

lon=alpha-ThetaG;                   %Calculating the Longitude
lat=Decl;                           %Assing the Latitude value
lon_deg=mod(lon,2*pi)./(pi).*180;
lat_deg=lat./(pi).*180;
Decl_deg=Decl/pi*180;
alpha_deg=alpha*180/pi;

== matlab function attitude_modela/Disturbance Torque/Solar Radiation Torque/Eclipse ==
  data: Sn input; y output; rr input
function y = eclipse(Sn, rr)

% Total eclipse model according to Wertz
%
% PROTOTYPE:
% out_eclipse = eclissi(Sn, rr, R_earth)
%
%---------------------------------INPUT------------------------------------
% sn = sun-earth distance [m]
% rr = position vector for compute the eclipse [km]
% R_earth = earth radius [km]
%
%-------------------------------OUTPUT-------------------------------------
% return a boolean variable:
% 0 : the SC is in shadow
% 1 : the SC is exposed to the sun
%  

Sn=Sn/1000; % convert in km
Rp = 6378; % Radius of Earth
Rs = 696340; % Radius of Sun
Sb = Sn-rr; 

S = norm(Sn);
C = Rp*S/(Rs-Rp);
Ds = norm(Sb);

Dp = norm(rr);
% rho_c = asin((Rs-Rp)/S);
rho_s = asin(Rs/Ds);
rho_p = asin(Rp/Dp);
theta = acos(dot(Sb/Ds,-rr/Dp));

y = ~(S<Ds && Ds<(S+C) && (rho_p-rho_s) > theta); % Eclipse Condition

% if (S<Ds && Ds<(S+C) && (rho_p-rho_s) > theta) %eclipse condition
%     y=0;
% else
%     y=1;
% end

== matlab function attitude_modela/Orbit Propagator/MATLAB Function ==
  data: a input; r_n output; e input; i input; OM input; om input; th input; R output
function [r_n, R] = par2rv(a, e, i, OM, om, th)
% function par2rv compute the position and velocity vector in cartesian coordinates from the
% coordinates from the keplerian parameters.
%
% PROTOTYPE
% 	[rr, vv] = par2rv(a, e, i ,OM, om, th)
%
%                 	---NOTATION---
%	-INPUT
% a = semi major axies [km]
% e = eccenticity
% i = inclination of orbital plane [rad]
% OM = right ascension of acending node [rad]
% om = anomaly of the periapsis [rad]
% th = true anomaly [rad]
%
%   -OUTPUT
% rr   	- position vector in cartesian coordinates
% vv   	- velocity vector in cartesian coordinates
%

%% INPUT control

if a<0
	error('a must be positive')
end
% if e<=0 || e>=1
% 	error('e must be in the interval [0,1]')
% end

%% position and velocity in perifocal frame
mu = 398600;
p = a*(1 - e^2);   b = sqrt(mu/p); 
R = p/(1 + e*cos(th)); % magnitude of position vector
 
% position vector in perifocal frame
rpf = [ R*cos(th); ...
    	 R*sin(th); ...
       	 0 ];

% velocity vector in perifocal frame
 vpf=[  -b*sin(th); ...
  	 b*(e+cos(th)); ...
       	 0  ];

OM=rad2deg(OM); om=rad2deg(om); i=rad2deg(i);
Rot =rotz(OM)*rotx(i)*rotz(om); % compute the rotation matrix

r_n=Rot*rpf;
%vv=Rot*vpf;

== matlab function attitude_modela/Orbit Propagator/Subsystem1/MATLAB Function ==
  data: theta input; Aln output; incl input; Om input; om input
function Aln = fcn(theta,incl,Om,om)
R_1=[cos(om+theta) sin(om+theta) 0;
    -sin(om+theta) cos(om+theta) 0;
    0 0 1];

R_2=[1 0 0; 
       0 cos(incl) sin(incl);
       0 -sin(incl) cos(incl)];
 
R_3=[ cos(Om) sin(Om) 0;
      -sin(Om) cos(Om) 0;
      0 0 1];
  
Aln=R_1*R_2*R_3;

== matlab function attitude_modela/Disturbance Torque/Magnetic Torque/Magnetic Field ==
  data: Sch input; r input; Br output; theta input; phi input; Bt output; Bp output
function [Br, Bt, Bp] = magnet(Sch, r, theta, phi)
% Inputs
%   r       Geocentric radius
%   theta   Latitude measured in degrees positive from equator
%   phi     Longitude measured in degrees positive east from Greenwich
%   days    Decimal days since January 1, 2000
%
% Outputs - magnetic field strength in local tangential coordinates
%   Br      B in radial direction%   Bt      B in theta direction
%   Bp      B in phi direction


% Checks to see if located at either pole to avoid singularities

if (theta>-0.00000001 && theta<0.00000001)
    theta=0.00000001;
elseif(theta<180.00000001 && theta>179.99999999)
    theta=179.99999999;
end
days = 500;

% The angles must be converted from degrees into radians

theta=(90-theta)*pi/180;
phi = phi*pi/180;

a=6371.2;  % Reference radius used in IGRF

% This section of the code simply reads in the g and h Schmidt
% quasi-normalized coefficients
gn=Sch.gn;
gm=Sch.gm;
gvali=Sch.gvali;
gsvi=Sch.gsvi;
hn=Sch.hn;
hm=Sch.hm;
hvali=Sch.hvali;
hsvi=Sch.hsvi;

N=max(gn);
g=zeros(N,N+1);
h=zeros(N,N+1);
for x=1:length(gn)
    g(gn(x),gm(x)+1) = gvali(x) + gsvi(x)*days/365;
    h(hn(x),hm(x)+1) = hvali(x) + hsvi(x)*days/365;
end

% Initialize each of the variables
% Br        B in the radial driection
% Bt        B in the theta direction12
% Bp        B in the phi direction
% P         The associated Legendre polynomial evaluated at cos(theta)
%           The nomenclature for the recursive values generally follows
%           the form P10 = P(n-1,m-0)
% dP        The partial derivative of P with respect to theta

Br=0;  Bt=0;  Bp=0;P11=1;
P10=P11;dP11=0;  dP10=dP11;
dP20=0;	P20=1;

for m=0:N
    for n=1:N
        if m<=n
            % Calculate Legendre polynomials and derivatives recursively
            if n==m
                P2 = sin(theta)*P11;
                dP2 = sin(theta)*dP11 + cos(theta)*P11;
                P11=P2;   P10=P11;   P20=0;
                dP11=dP2; dP10=dP11; dP20=0;
            elseif n==1
                P2 = cos(theta)*P10;
                dP2 = cos(theta)*dP10 - sin(theta)*P10;
                P20=P10;   P10=P2;
                dP20=dP10; dP10=dP2;
            else
                K = ((n-1)^2-m^2)/((2*n-1)*(2*n-3));
                P2 = cos(theta)*P10 - K*P20;
                dP2 = cos(theta)*dP10 - sin(theta)*P10 - K*dP20;
                P20=P10;   P10=P2;
                dP20=dP10; dP10=dP2;
            end
            
            % Calculate Br, Bt, and Bp
            Br = Br + (a/r)^(n+2)*(n+1)*...
                ((g(n,m+1)*cos(m*phi) + h(n,m+1)*sin(m*phi))*P2);
            Bt = Bt + (a/r)^(n+2)*...
                ((g(n,m+1)*cos(m*phi) + h(n,m+1)*sin(m*phi))*dP2);
            Bp = Bp + (a/r)^(n+2)*...
                (m*(-g(n,m+1)*sin(m*phi) + h(n,m+1)*cos(m*phi))* P2);
        end
    end
end

Br=Br;
Bt=-Bt;
Bp=-Bp/sin(theta);

== matlab function attitude_modela/Disturbance Torque/Drag Torque/Drag Torque ==
  data: Abn input; Mdrag output; par input; theta input
function Mdrag = atmospheric_drag_torque(Abn, par, theta)

% assumption: the pressure centre is the the geometric centre of the
% surfaces of the satellite

% parameters
Cd = 2.2;    % parameter from experiments

% [km kg/m^3 km]
rho_table = [0 1.225 7.249 ;
    25 3.899e-2 6.349 ;
    30 1.774e-2 6.682 ;
    40 3.972e-3 7.554 ;
    50 1.057e-3 8.382 ;
    60 3.206e-4 7.714 ;
    70 8.770e-5 6.549 ;
    80 1.905e-5 5.779 ;
    90 3.396e-6 5.382 ;
    100 5.297e-7 5.877 ;
    110 9.661e-8 7.263 ;
    120 2.438e-8 9.473 ;
    130 8.484e-9 12.636 ;
    140 3.845e-9 16.149 ;
    150 2.070e-9 22.523 ;
    180 5.464e-10 29.740 ;
    200 2.789e-10 37.105 ;
    250 7.248e-11 45.548 ;
    300 2.418e-11 53.628 ;
    350 9.158e-12 53.298 ;
    400 3.725e-12 58.515 ;
    450 1.585e-12 60.828 ;
    500 6.967e-13 63.822 ;
    600 1.454e-13 71.835 ;
    700 3.614e-14 88.667 ;
    800 1.170e-14 124.64 ;
    900 5.245e-15 181.05 ;
    1000 3.019e-15 268.00];

mu = 398600;
a = par(1); % semimajor axis [km]
e = par(2); % eccentricity
p = a*(1-e^2); % semilatum rectum [km]
r = p/(1+e*cos(theta)); % distance from focus in km
earth_radius = 6.3781e+3; %[km] %correction, before it was e+6
h = r - earth_radius; %[km]
% R = sqrt(r^2+(e*a)^2+2*r*e*a*cos(theta)) % distance from earth

%selection of rho_
select = 0;

for ind = 2:28
    if h < rho_table(ind,1)
        select = ind - 1;
        break
    end
end

if select == 0
    select = 28;
end

h_0     =   rho_table(select, 1);
rho_0   =   rho_table(select, 2);
H       =   rho_table(select, 3);
rho_ = rho_0*exp(-(h-h_0)/H);

Rpf = r*[cos(theta) sin(theta) 0]'*1e+3; % perifocal ray in meters
Vpf = sqrt(mu/p)*1e+3*[-sin(theta) e+cos(theta) 0]'; % perifocal speed

dec = zeros(6,1);

A = [6 2 3 6 2 3]'*1e-2;
F = zeros(3,6);
Mdrag = [0 0 0]';

r__ = [0.1 0 0;
    0 0.3 0;
    0 0 0.2;
    -0.1 0 0;
    0 -0.3 0;
    0 0 -0.2]';

ldir = [eye(3) -eye(3)];

% check whether to calculate Mi

i = par(3);
OM = par(4);
w = par(5);

ci = cos(i);
si = sin(i);
cw = cos(w);
sw = sin(w);
cO = cos(OM);
sO = sin(OM);

A313 = [cw*cO-sw*sO*ci cw*sO+sw*cO*ci sw*si;
    -sw*cO-cw*sO*ci -sw*sO+cw*cO*ci cw*si;
    sO*si -cO*si cO];

N = A313*ldir;

% r in earth centred inertial reference system
r_ECI = A313'*Rpf;
v_ECI = A313'*Vpf;

w_e = 2*pi/(23*3600+56*60+4.09);
% -rxw = +wxr
v_r = Abn * (v_ECI+cross([0 0 w_e]',r_ECI));



% if the scalar product between n and v_r is positive then we calculate the
% drag force
for i = 1 : 6
    if N(:,i)'*v_r > 0
        % save index
        dec(i) = 1;
    end
end

% calculate Fi and M

for ind = 1 : 6
    if dec(ind) == 1 
        F(:,ind) = -Cd/2*rho_*(v_r'*v_r)*v_r/norm(v_r,2)*(N(:,ind)'*v_r/norm(v_r,2))*A(ind);
    end
    Mdrag = Mdrag + cross(r__(:,ind),F(:,ind));
end

== matlab function attitude_modela/Subsystem1/sens ==
  data: BN input; barBN output; s_N input; m_N input
function barBN = direction_cosines_estimation(BN, s_N, m_N)


% BN real direction cosines matrix 3x3
% s_N known vector 3x1 pointing to the sun in the earth reference frame,
% s_N know vector 3x1 pointing as the magnetic field in earth reference
% frame


% real vectors
s_B_true = BN*s_N;
m_B_true = BN*m_N;

% adding noise
s_B = s_B_true + (rand([3,1])-0.5)/5/10;
m_B = m_B_true + (rand([3,1])-0.5)/5; % noise might depend on altitude

% normalization
s_B = s_B/norm(s_B);
m_B = m_B/norm(m_B);

% triad method
t1_B = s_B;
t2_B = cross(s_B,m_B)/norm(cross(s_B,m_B));
t3_B = cross(t1_B,t2_B);

t1_N = s_N/norm(s_N);
t2_N = cross(s_N,m_N)/norm(cross(s_N,m_N));
t3_N = cross(t1_N,t2_N);

barBT = [t1_B t2_B t3_B];
NT = [t1_N t2_N t3_N];

barBN = barBT*NT';

barBB = barBN*BN';

%accuracy = acos(0.5*(trace(barBB)-1))*180/pi; % error in degrees;

== matlab function attitude_modela/Disturbance Torque/Solar Radiation Torque/If Action Subsystem/Torque Compute ==
  data: Sb input; Mspr output; solar_par input
function Mspr = torque_compute(Sb, solar_par)

% Parameters
Ab = solar_par.Ab;
nb = solar_par.nb;
rhosb = solar_par.rhosb;
rhodb = solar_par.rhodb;
rb = solar_par.rb;
As = solar_par.As;
ns = solar_par.ns;
rhosp = solar_par.rhosp;
rhodp = solar_par.rhodp;
rp = solar_par.rp;
xg = solar_par.xg;

Fe=1358; %[W/m^2]
c=3*10^8; %[m/s]
P=Fe/c; %[N/m^2]
%sb=[sb1; sb2; sb3];

f=zeros(3,10);
T=zeros(3,10);
 
Mspr=[0;0;0];

for i=1:length(nb)
    f=-P*Ab(i)*(dot(Sb,nb(:,i)))*((1-rhosb)*Sb+(2*rhosb*dot(Sb,nb(:,i))+2/3*rhodb)*nb(:,i));
    T(:,i)=cross(rb(:,i)-xg,f)*(dot(Sb,nb(:,i))>=0);

    Mspr=Mspr+T(:,i);
end
for j=1:length(ns)
    f=-P*As(j)*(dot(Sb,ns(:,j)))*((1-rhosp)*Sb+(2*rhosp*dot(Sb,ns(:,j))+2/3*rhodp)*ns(:,j));
    T(:,j)=cross(rp(:,j)-xg,f)*(dot(Sb,ns(:,j))>=0);

    Mspr=Mspr+T(:,j); %[kg*m^2/s^2]
end

== matlab function attitude_modela/MATLAB Function1 ==
  data: var input; out output
function out = angular_noise(var)
dev = sqrt(var);
y = dev*randn([3,1]); % gaussian noise with zero mean

== matlab function attitude_modela/MATLAB Function2 ==
  data: var input; out output
function out = angular_noise(var)
dev = sqrt(var);
y = dev*randn([3,1]); % gaussian noise with zero mean

== matlab function attitude_modela/Subsystem1/from rotation matrix to euler angles1 ==
  data: Abn input; eul output
function eul = Abn2Euler(Abn)
alpha = atan2(Abn(1,3),Abn(2,3)) + pi;
beta = atan2(Abn(1,3)/sin(alpha), Abn(3,3));
gamma = atan2(Abn(3,1),Abn(3,2));
eul = [alpha beta gamma]';
eul = eul*180/pi;

== matlab function attitude_modela/Subsystem1/MATLAB Function ==
  data: Abn input; e output
function e = ang(Abn)
% phi = acos(0.5*trace(Abn)-0.5);
% %e = [(Abn(2,3)-Abn(3,2))/2*sin(phi) (Abn(3,1)-Abn(1,3))/2*sin(phi) (Abn(1,2)-Abn(2,1))/2*sin(phi)]';
%e = [acos(Abn(3,3)) atan2(Abn(3,1),Abn(3,2)) atan2(Abn(1,3),Abn(2,3))]';
e = rotm2eul(Abn,'ZYZ');

== matlab function attitude_modela/Disturbance Torque/Magnetic Torque/Local2Geoc ==
  data: Br input; Bx output; Bt input; Bp input; lat input; LST input; By output; Bz output
function [Bx,By,Bz] = LocalTangen2Geocetric(Br,Bt,Bp,lat,LST)
% Inputs
%   Br      B in radial direction   | Magnetic field strength (B)
%   Bt      B in theta direction    | in local tangential coordinates
%   Bp      B in phi direction      |
%   LST     Local sidereal time of location (degrees)
%   lat     Latitude measured positive north from equator (degrees) 
% Outputs
%   Bx      B in x-direction        | Magnetic field strength (B)
%   By      B in y-direction        | in geocentric inertial coordinates
%   Bz      B in z-direction        |

lat=lat*pi/180;
LST=LST*pi/180;
% Coordinate transformation

Bx = (Br*cos(lat)+Bt*sin(lat))*cos(LST) - Bp*sin(LST);
By = (Br*cos(lat)+Bt*sin(lat))*sin(LST) + Bp*cos(LST);
Bz = (Br*sin(lat)+Bt*cos(lat));
